simulink library "hc12drivers"  (Simulink 6.0)
settings: Solver=ode45  SolverMode=SingleTasking  StartTime=0.0  StopTime=10.0  RelTol=1e-3
undefined symbols (not defined in the file or in its folder): hc12_hminit
settings Model: Creator=jims  LastModifiedBy=jcarrick  ProdHWDeviceType=Specified  Master=hc12drivers/Master
settings DataIOCC: SignalLoggingName=logsOut
settings OptimizationCC: BooleanDataType=off
settings DebuggingCC: CheckExecutionContextPreStartOutputMsg=on  CheckExecutionContextRuntimeOutputMsg=on  SolverPrmCheckMsg=none
settings HardwareCC: ProdHWDeviceType=Specified
settings GRTTargetCC: LifeSpan=inf
settings SFSimCC: SFSimApplyToAllLibs=on  SFSimBuildMode=Incremental

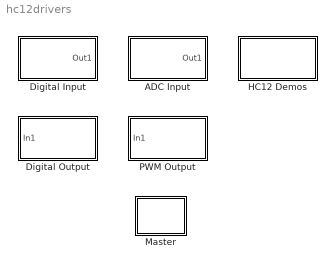
== system hc12drivers ==
  ADC Input : Subsystem  EnableExecutionContextPropagation=on  mask{bank=0, channels=[1 2], use10bits=8 bits, left_justify=Right justified, sampletime=0.065536}
      mask prompts: bank "ADC bank:"; channels "Channels ( 0 - 7 ):"; use10bits "ADC resolution:"; left_justify "Word alignment:"; sampletime "Sample time:"
      mask help:
      | The ADC Input block reads up to 8 channels of data from one of two
      | 8-channel analog-to-digital converter (ADC) banks.
      mask init:
      | hc12_adc_v_mcb(bank-1);
      mask Help: helpview([docroot '/toolbox/hc12/hc12.map'],'hc12_ADC_In_blkref')
      mask StyleString: popup(0|1),edit,popup(8 bits|10 bits),popup(Right justified|Left justified),edit
      mask Display: disp('ADC Input')
  Digital Input : Subsystem  EnableExecutionContextPropagation=on  mask{diport=A}
      mask prompts: diport "Input port"
      mask help: Specify the port (A or B) used for input.
      mask init:
      | hc12_di_abbyte_mcb(diport)
      mask Help: helpview([docroot '/toolbox/hc12/hc12.map'],'hc12_Digital_In_blkref')
      mask StyleString: popup(A|B)
      mask Display: disp('PORT A or B')
  Digital Output : Subsystem  EnableExecutionContextPropagation=on  mask{doport=B}
      mask prompts: doport "Output port"
      mask help: Specify the port (A or B) used for output.
      mask init:
      | hc12_do_abbyte_mcb(doport)
      mask Help: helpview([docroot '/toolbox/hc12/hc12.map'],'hc12_Digital_Out_blkref')
      mask StyleString: popup(A|B)
      mask Display: disp('PORT A or B')
  HC12 Demos : Subsystem  EnableExecutionContextPropagation=on
      mask Display: disp('Demos')
  Master : Subsystem  Tag=HardwareResourceMaster  Priority=100  LoadFcn=hc12_hminit;  InitFcn=hc12_hminit;  StartFcn=hc12_hminit;  EnableExecutionContextPropagation=on  mask{osc=16000000, desiredST=0.065536}
      mask prompts: osc "Clock frequency:"; desiredST "Sample time:"
      mask help:
      | The Master block provides the following core functionality for the model:
      |
      |   Sets the real-time clock period on the HC12. See Setting HC12 Timing Parameters.
      |
      |   Manages a resource database to arbitrate potentially conflicting requests for HC12
      |   hardware resources (such as ports) by device driver blocks.
      mask init:
      | % HC12 resource object.
      | %
      | % Derive base sample time from osc
      | % and desiredST in the Master block.
      | %
      | % Then, determine the achievable
      | % sample time and set the values of the
      | % CRG RTR values: RTR30 and RTR64
      | % for the HC12.
      | 
      | hc12_master_mcb(desiredST, osc);
      settings: CopyFcn=hc12_hminit;  OpenFcn=hc12_hminit;open_system(gcb,'mask')
      settings: DeleteFcn=|
      | if isappdata(0,'hc12driversMaster')
      |    rmappdata(0,'hc12driversMaster');
      | end
      mask Help: helpview([docroot '/toolbox/hc12/hc12.map'],'hc12_Master_blkref')
      mask Display: image(imread('target_icon.jpg'))
  PWM Output : Subsystem  EnableExecutionContextPropagation=on  mask{channel=0, polaritybit=off, clkbit=off, caebit=off, pwmper=255}
      mask prompts: channel "PWM channel:"; polaritybit "Invert polarity"; clkbit "PWMCLK  (unchecked = clock [A, B];   checked = clock [SA, SB])"; caebit "Center aligned (unchecked = left aligned)"; pwmper "PWM period:"
      mask help:
      | The block input signal specifies the PWM duty cycle register value PWMDTYx in raw units ranging from 0 to 255.
      |
      | PWMPERx is specified in the PWM period dialog below. Duty cycle is determined by the following expression:
      | Duty Cycle = 100 * (PWMPERx - PWMDTYx) / PWMPERx
      |
      | In the generated code, the input signal PWMDTYx is limited not to exceed PWMPERx which would otherwise result in a sign change in the equation above.
      |
      | Note:
      | PWMCLK A or SA used for channels 0, 1, 4, 5
      | PWMCLK B or SB used for channels 2, 3, 6, 7
      mask init:
      | hc12_pwm_mcb(channel)
      mask Help: helpview([docroot '/toolbox/hc12/hc12.map'],'hc12_PWM_Out_blkref')
      mask StyleString: popup(0|1|2|3|4|5|6|7),checkbox,checkbox,checkbox,edit
      mask Display: disp('PWM Output')

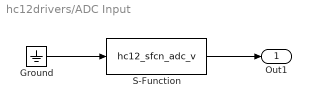
== system hc12drivers/ADC Input ==
  Ground : Ground
  S-Function : S-Function  FunctionName=hc12_sfcn_adc_v  Parameters=uint8(bank-1), uint16(channels), uint8(use10bits-1), uint8(left_justify-1), sampletime
  Out1 : Outport
  wires:
  Ground/1 -> S-Function/1
  S-Function/1 -> Out1/1

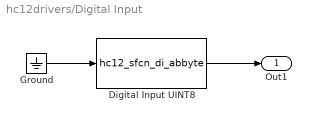
== system hc12drivers/Digital Input ==
  Digital Input UINT8 : S-Function  Tag=HC12DriverData  FunctionName=hc12_sfcn_di_abbyte
  Ground : Ground
  Out1 : Outport
  wires:
  Ground/1 -> Digital Input UINT8/1
  Digital Input UINT8/1 -> Out1/1

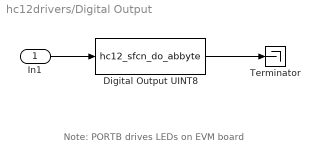
== system hc12drivers/Digital Output ==
  note: Note: PORTB drives LEDs on EVM board
  In1 : Inport  LatchInput=off
  Digital Output UINT8 : S-Function  Tag=HC12DriverData  FunctionName=hc12_sfcn_do_abbyte
  Terminator : Terminator
  wires:
  Digital Output UINT8/1 -> Terminator/1
  In1/1 -> Digital Output UINT8/1

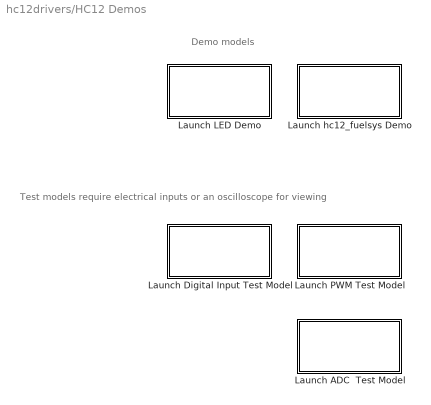
== system hc12drivers/HC12 Demos ==
  note: Test models require electrical inputs
      | or an oscilloscope for viewing
  note: Demo models
  Launch ADC  Test Model : Subsystem  EnableExecutionContextPropagation=on  mask{A=}
      mask prompts: A "Needed to invoke correct OpenFcn from Browser:"
      settings: OpenFcn=open_system('hc12_adc');
      mask Display: disp('ADC Test Model')
  Launch Digital Input Test Model : Subsystem  EnableExecutionContextPropagation=on  mask{A=}
      mask prompts: A "Needed to invoke correct OpenFcn from Browser:"
      settings: OpenFcn=open_system('hc12_di');
      mask Display: disp('Digital Input\nTest Model')
  Launch LED Demo : Subsystem  EnableExecutionContextPropagation=on  mask{A=}
      mask prompts: A "Needed to invoke correct OpenFcn from Browser:"
      settings: OpenFcn=open_system('hc12_led');
      mask Display: disp('LED Demo')
  Launch PWM Test Model : Subsystem  EnableExecutionContextPropagation=on  mask{A=}
      mask prompts: A "Needed to invoke correct OpenFcn from Browser:"
      settings: OpenFcn=open_system('hc12_pwm');
      mask Display: disp('PWM Test Model')
  Launch hc12_fuelsys Demo : Subsystem  EnableExecutionContextPropagation=on  mask{A=}
      mask prompts: A "Needed to invoke correct OpenFcn from Browser:"
      settings: OpenFcn=open_system('hc12_fuelsys');
      mask Display: disp('hc12_fuelsys Demo')

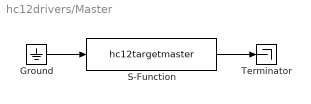
== system hc12drivers/Master ==
  Ground : Ground
  S-Function : S-Function  Tag=HC12DriverData  FunctionName=hc12targetmaster
  Terminator : Terminator
  wires:
  S-Function/1 -> Terminator/1
  Ground/1 -> S-Function/1

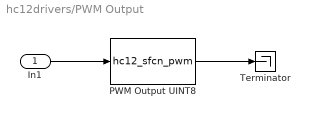
== system hc12drivers/PWM Output ==
  In1 : Inport  LatchInput=off
  PWM Output UINT8 : S-Function  Tag=HC12DriverData  FunctionName=hc12_sfcn_pwm  Parameters=boolean(polaritybit), boolean(clkbit), boolean(caebit), uint8(pwmper)
  Terminator : Terminator
  wires:
  In1/1 -> PWM Output UINT8/1
  PWM Output UINT8/1 -> Terminator/1

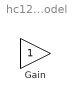
== system hc12drivers/HC12 Demos/Launch ADC  Test Model ==
  Gain : Gain  SaturateOnIntegerOverflow=on

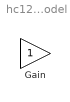
== system hc12drivers/HC12 Demos/Launch Digital Input Test Model ==
  Gain : Gain  SaturateOnIntegerOverflow=on

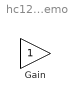
== system hc12drivers/HC12 Demos/Launch LED Demo ==
  Gain : Gain  SaturateOnIntegerOverflow=on

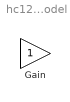
== system hc12drivers/HC12 Demos/Launch PWM Test Model ==
  Gain : Gain  SaturateOnIntegerOverflow=on

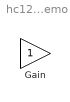
== system hc12drivers/HC12 Demos/Launch hc12_fuelsys Demo ==
  Gain : Gain  SaturateOnIntegerOverflow=on
